simulink model "MCK_system"  (R2020b)
settings: Solver=VariableStepAuto  StartTime=0.0  StopTime=200  RelTol=1e-3
settings Model: Creator=jjw05  LastModifiedBy=jjw05

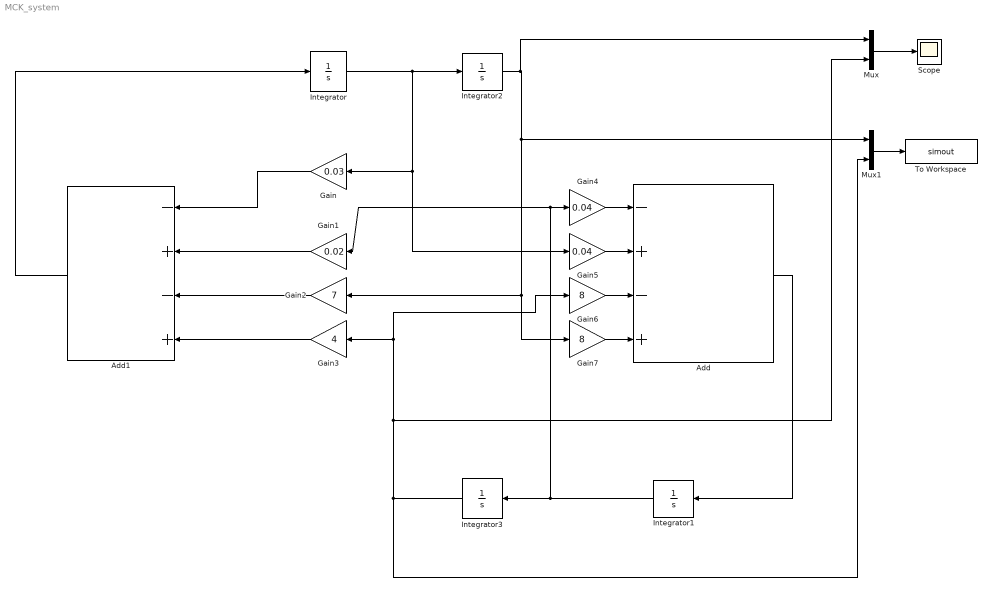
== system MCK_system ==
  Add : Sum  Inputs=-+-+
  Add1 : Sum  Inputs=-+-+
  Gain : Gain  Gain=0.03
  Gain1 : Gain  Gain=0.02
  Gain2 : Gain  Gain=7
  Gain3 : Gain  Gain=4
  Gain4 : Gain  Gain=0.04
  Gain5 : Gain  Gain=0.04
  Gain6 : Gain  Gain=8
  Gain7 : Gain  Gain=8
  Integrator : Integrator
  Integrator1 : Integrator
  Integrator2 : Integrator
  Integrator3 : Integrator  InitialCondition=1
  Mux : Mux  Inputs=2
  Mux1 : Mux  Inputs=2
  Scope : Scope
  To Workspace : ToWorkspace  VariableName=simout  SaveFormat=Timeseries  SampleTime=-1
  wires:
  Gain/1 -> Add1/1
  Integrator/1 -> Integrator2/1, Gain5/1, Gain/1
  Add1/1 -> Integrator/1
  Add/1 -> Integrator1/1
  Integrator1/1 -> Gain4/1, Gain1/1, Integrator3/1
  Gain1/1 -> Add1/2
  Integrator2/1 -> Mux1/1, Gain7/1, Gain2/1, Mux/1
  Gain2/1 -> Add1/3
  Gain3/1 -> Add1/4
  Integrator3/1 -> Gain6/1, Gain3/1, Mux/2, Mux1/2
  Gain4/1 -> Add/1
  Gain5/1 -> Add/2
  Gain6/1 -> Add/3
  Gain7/1 -> Add/4
  Mux/1 -> Scope/1
  Mux1/1 -> To Workspace/1
